simulink model "GalacticSoupFunctional"  (R2025b)
settings: Solver=VariableStepAuto  StartTime=0.0  StopTime=10.0  RelTol=1e-3
settings Model: DataDictionary=GalacticSoupFunctionalInterfaces.sldd  Creator=sarah  LastModifiedBy=sarah

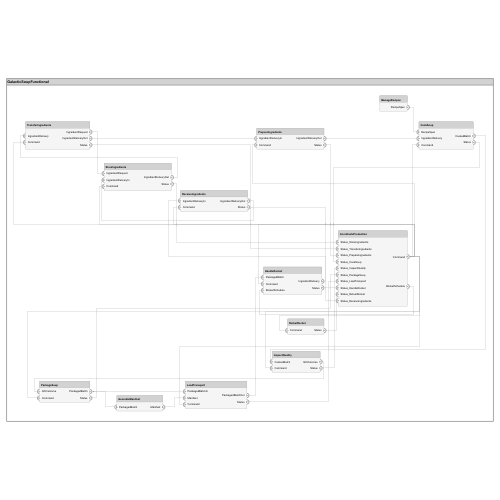
[thumbnail: Simulink's stored preview of the top-level diagram]
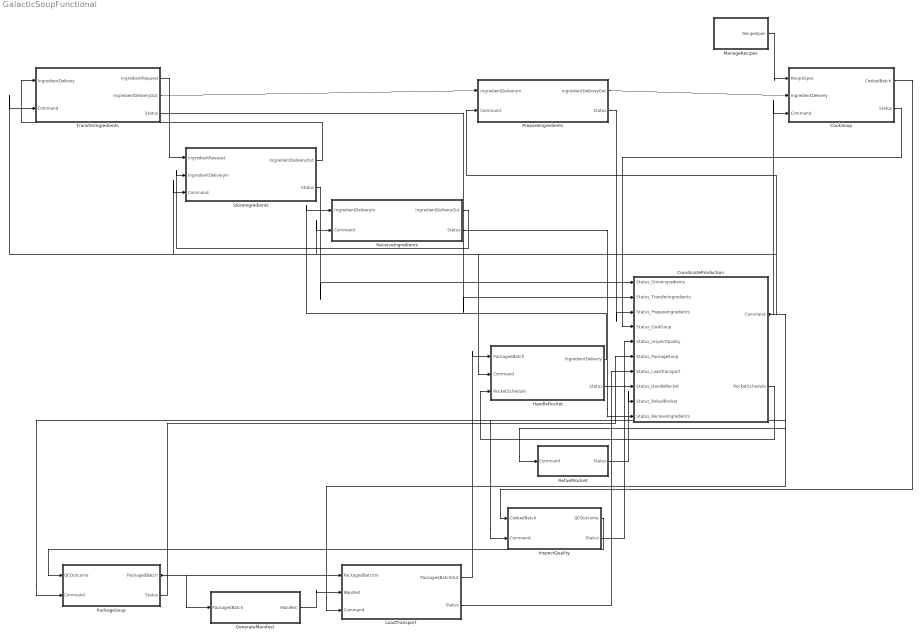
== system GalacticSoupFunctional ==
  CookSoup : Subsystem
      settings: PortSchema="{\"entries\":[{\"content\":{\"headerSize\":26,\"margin\":15,\"minimumSpacing\":25,\"sides\":[{\"content\":{\"connectorIds\":[\"In1\",\"In2\",\"In3\"]},\"type\":\"ConnectorPlacement.EquallySpacedRectSide\",\"uuid\":\"47548036-a6c3-440f-b573-2a4e753e82ae\"},{\"content\":{\"connectorIds\":[\"Out1\",\"Out2\"],\"side\":\"RIGHT\"},\"type\":\"ConnectorPlacement.EquallySpacedRectSide\",\"uuid\":\"ab096620-2054-4429-8520-52cfe6541bb8\"},{\"content\":{\"side\":\"TOP\"},\"type\":\"ConnectorPlacement.EquallySpacedRectSide\",\"uuid\":\"6e18e29c-ba68-48ca-8847-f496b38e15b5\"}]},\"type\":\"ConnectorPlacement.EquallySpacedConnector\",\"uuid\":\"7233fc04-a641-40d9-8870-909b934a9733\"}],\"packageUris\":[\"http://schema.mathworks.com/mf0/Connector/R2020b\"],\"version\":\"1.0\"}"
  CoordinateProduction : Subsystem
      settings: PortSchema="{\"entries\":[{\"content\":{\"headerSize\":26,\"margin\":15,\"minimumSpacing\":25,\"sides\":[{\"content\":{\"connectorIds\":[\"In1\",\"In2\",\"In3\",\"In4\",\"In5\",\"In6\",\"In7\",\"In8\",\"In9\",\"In10\"]},\"type\":\"ConnectorPlacement.EquallySpacedRectSide\",\"uuid\":\"47548036-a6c3-440f-b573-2a4e753e82ae\"},{\"content\":{\"connectorIds\":[\"Out1\",\"Out2\"],\"side\":\"RIGHT\"},\"type\":\"ConnectorPlacement.EquallySpacedRectSide\",\"uuid\":\"ab096620-2054-4429-8520-52cfe6541bb8\"},{\"content\":{\"side\":\"TOP\"},\"type\":\"ConnectorPlacement.EquallySpacedRectSide\",\"uuid\":\"6e18e29c-ba68-48ca-8847-f496b38e15b5\"}]},\"type\":\"ConnectorPlacement.EquallySpacedConnector\",\"uuid\":\"7233fc04-a641-40d9-8870-909b934a9733\"}],\"packageUris\":[\"http://schema.mathworks.com/mf0/Connector/R2020b\"],\"version\":\"1.0\"}"
  GenerateManifest : Subsystem
      settings: PortSchema="{\"entries\":[{\"content\":{\"headerSize\":26,\"margin\":15,\"minimumSpacing\":25,\"sides\":[{\"content\":{\"connectorIds\":[\"In1\"]},\"type\":\"ConnectorPlacement.EquallySpacedRectSide\",\"uuid\":\"47548036-a6c3-440f-b573-2a4e753e82ae\"},{\"content\":{\"connectorIds\":[\"Out1\"],\"side\":\"RIGHT\"},\"type\":\"ConnectorPlacement.EquallySpacedRectSide\",\"uuid\":\"ab096620-2054-4429-8520-52cfe6541bb8\"},{\"content\":{\"side\":\"TOP\"},\"type\":\"ConnectorPlacement.EquallySpacedRectSide\",\"uuid\":\"6e18e29c-ba68-48ca-8847-f496b38e15b5\"}]},\"type\":\"ConnectorPlacement.EquallySpacedConnector\",\"uuid\":\"7233fc04-a641-40d9-8870-909b934a9733\"}],\"packageUris\":[\"http://schema.mathworks.com/mf0/Connector/R2020b\"],\"version\":\"1.0\"}"
  HandleRocket : Subsystem
      settings: PortSchema="{\"entries\":[{\"content\":{\"headerSize\":26,\"margin\":15,\"minimumSpacing\":25,\"sides\":[{\"content\":{\"connectorIds\":[\"In1\",\"In2\",\"In3\"]},\"type\":\"ConnectorPlacement.EquallySpacedRectSide\",\"uuid\":\"47548036-a6c3-440f-b573-2a4e753e82ae\"},{\"content\":{\"connectorIds\":[\"Out1\",\"Out2\"],\"side\":\"RIGHT\"},\"type\":\"ConnectorPlacement.EquallySpacedRectSide\",\"uuid\":\"ab096620-2054-4429-8520-52cfe6541bb8\"},{\"content\":{\"side\":\"TOP\"},\"type\":\"ConnectorPlacement.EquallySpacedRectSide\",\"uuid\":\"6e18e29c-ba68-48ca-8847-f496b38e15b5\"}]},\"type\":\"ConnectorPlacement.EquallySpacedConnector\",\"uuid\":\"7233fc04-a641-40d9-8870-909b934a9733\"}],\"packageUris\":[\"http://schema.mathworks.com/mf0/Connector/R2020b\"],\"version\":\"1.0\"}"
  InspectQuality : Subsystem
      settings: PortSchema="{\"entries\":[{\"content\":{\"headerSize\":26,\"margin\":15,\"minimumSpacing\":25,\"sides\":[{\"content\":{\"connectorIds\":[\"In1\",\"In2\"]},\"type\":\"ConnectorPlacement.EquallySpacedRectSide\",\"uuid\":\"47548036-a6c3-440f-b573-2a4e753e82ae\"},{\"content\":{\"connectorIds\":[\"Out1\",\"Out2\"],\"side\":\"RIGHT\"},\"type\":\"ConnectorPlacement.EquallySpacedRectSide\",\"uuid\":\"ab096620-2054-4429-8520-52cfe6541bb8\"},{\"content\":{\"side\":\"TOP\"},\"type\":\"ConnectorPlacement.EquallySpacedRectSide\",\"uuid\":\"6e18e29c-ba68-48ca-8847-f496b38e15b5\"}]},\"type\":\"ConnectorPlacement.EquallySpacedConnector\",\"uuid\":\"7233fc04-a641-40d9-8870-909b934a9733\"}],\"packageUris\":[\"http://schema.mathworks.com/mf0/Connector/R2020b\"],\"version\":\"1.0\"}"
  LoadTransport : Subsystem
      settings: PortSchema="{\"entries\":[{\"content\":{\"headerSize\":26,\"margin\":15,\"minimumSpacing\":25,\"sides\":[{\"content\":{\"connectorIds\":[\"In1\",\"In2\",\"In3\"]},\"type\":\"ConnectorPlacement.EquallySpacedRectSide\",\"uuid\":\"47548036-a6c3-440f-b573-2a4e753e82ae\"},{\"content\":{\"connectorIds\":[\"Out1\",\"Out2\"],\"side\":\"RIGHT\"},\"type\":\"ConnectorPlacement.EquallySpacedRectSide\",\"uuid\":\"ab096620-2054-4429-8520-52cfe6541bb8\"},{\"content\":{\"side\":\"TOP\"},\"type\":\"ConnectorPlacement.EquallySpacedRectSide\",\"uuid\":\"6e18e29c-ba68-48ca-8847-f496b38e15b5\"}]},\"type\":\"ConnectorPlacement.EquallySpacedConnector\",\"uuid\":\"7233fc04-a641-40d9-8870-909b934a9733\"}],\"packageUris\":[\"http://schema.mathworks.com/mf0/Connector/R2020b\"],\"version\":\"1.0\"}"
  ManageRecipes : Subsystem
      settings: PortSchema="{\"entries\":[{\"content\":{\"headerSize\":26,\"margin\":15,\"minimumSpacing\":25,\"sides\":[{\"content\":{},\"type\":\"ConnectorPlacement.EquallySpacedRectSide\",\"uuid\":\"47548036-a6c3-440f-b573-2a4e753e82ae\"},{\"content\":{\"connectorIds\":[\"Out1\"],\"side\":\"RIGHT\"},\"type\":\"ConnectorPlacement.EquallySpacedRectSide\",\"uuid\":\"ab096620-2054-4429-8520-52cfe6541bb8\"},{\"content\":{\"side\":\"TOP\"},\"type\":\"ConnectorPlacement.EquallySpacedRectSide\",\"uuid\":\"6e18e29c-ba68-48ca-8847-f496b38e15b5\"}]},\"type\":\"ConnectorPlacement.EquallySpacedConnector\",\"uuid\":\"7233fc04-a641-40d9-8870-909b934a9733\"}],\"packageUris\":[\"http://schema.mathworks.com/mf0/Connector/R2020b\"],\"version\":\"1.0\"}"
  PackageSoup : Subsystem
      settings: PortSchema="{\"entries\":[{\"content\":{\"headerSize\":26,\"margin\":15,\"minimumSpacing\":25,\"sides\":[{\"content\":{\"connectorIds\":[\"In1\",\"In2\"]},\"type\":\"ConnectorPlacement.EquallySpacedRectSide\",\"uuid\":\"47548036-a6c3-440f-b573-2a4e753e82ae\"},{\"content\":{\"connectorIds\":[\"Out1\",\"Out2\"],\"side\":\"RIGHT\"},\"type\":\"ConnectorPlacement.EquallySpacedRectSide\",\"uuid\":\"ab096620-2054-4429-8520-52cfe6541bb8\"},{\"content\":{\"side\":\"TOP\"},\"type\":\"ConnectorPlacement.EquallySpacedRectSide\",\"uuid\":\"6e18e29c-ba68-48ca-8847-f496b38e15b5\"}]},\"type\":\"ConnectorPlacement.EquallySpacedConnector\",\"uuid\":\"7233fc04-a641-40d9-8870-909b934a9733\"}],\"packageUris\":[\"http://schema.mathworks.com/mf0/Connector/R2020b\"],\"version\":\"1.0\"}"
  PrepareIngredients : Subsystem
      settings: PortSchema="{\"entries\":[{\"content\":{\"headerSize\":26,\"margin\":15,\"minimumSpacing\":25,\"sides\":[{\"content\":{\"connectorIds\":[\"In1\",\"In2\"]},\"type\":\"ConnectorPlacement.EquallySpacedRectSide\",\"uuid\":\"47548036-a6c3-440f-b573-2a4e753e82ae\"},{\"content\":{\"connectorIds\":[\"Out1\",\"Out2\"],\"side\":\"RIGHT\"},\"type\":\"ConnectorPlacement.EquallySpacedRectSide\",\"uuid\":\"ab096620-2054-4429-8520-52cfe6541bb8\"},{\"content\":{\"side\":\"TOP\"},\"type\":\"ConnectorPlacement.EquallySpacedRectSide\",\"uuid\":\"6e18e29c-ba68-48ca-8847-f496b38e15b5\"}]},\"type\":\"ConnectorPlacement.EquallySpacedConnector\",\"uuid\":\"7233fc04-a641-40d9-8870-909b934a9733\"}],\"packageUris\":[\"http://schema.mathworks.com/mf0/Connector/R2020b\"],\"version\":\"1.0\"}"
  ReceiveIngredients : Subsystem
      settings: PortSchema="{\"entries\":[{\"content\":{\"headerSize\":26,\"margin\":15,\"minimumSpacing\":25,\"sides\":[{\"content\":{\"connectorIds\":[\"In1\",\"In2\"]},\"type\":\"ConnectorPlacement.EquallySpacedRectSide\",\"uuid\":\"47548036-a6c3-440f-b573-2a4e753e82ae\"},{\"content\":{\"connectorIds\":[\"Out1\",\"Out2\"],\"side\":\"RIGHT\"},\"type\":\"ConnectorPlacement.EquallySpacedRectSide\",\"uuid\":\"ab096620-2054-4429-8520-52cfe6541bb8\"},{\"content\":{\"side\":\"TOP\"},\"type\":\"ConnectorPlacement.EquallySpacedRectSide\",\"uuid\":\"6e18e29c-ba68-48ca-8847-f496b38e15b5\"}]},\"type\":\"ConnectorPlacement.EquallySpacedConnector\",\"uuid\":\"7233fc04-a641-40d9-8870-909b934a9733\"}],\"packageUris\":[\"http://schema.mathworks.com/mf0/Connector/R2020b\"],\"version\":\"1.0\"}"
  RefuelRocket : Subsystem
      settings: PortSchema="{\"entries\":[{\"content\":{\"headerSize\":26,\"margin\":15,\"minimumSpacing\":25,\"sides\":[{\"content\":{\"connectorIds\":[\"In1\"]},\"type\":\"ConnectorPlacement.EquallySpacedRectSide\",\"uuid\":\"47548036-a6c3-440f-b573-2a4e753e82ae\"},{\"content\":{\"connectorIds\":[\"Out1\"],\"side\":\"RIGHT\"},\"type\":\"ConnectorPlacement.EquallySpacedRectSide\",\"uuid\":\"ab096620-2054-4429-8520-52cfe6541bb8\"},{\"content\":{\"side\":\"TOP\"},\"type\":\"ConnectorPlacement.EquallySpacedRectSide\",\"uuid\":\"6e18e29c-ba68-48ca-8847-f496b38e15b5\"}]},\"type\":\"ConnectorPlacement.EquallySpacedConnector\",\"uuid\":\"7233fc04-a641-40d9-8870-909b934a9733\"}],\"packageUris\":[\"http://schema.mathworks.com/mf0/Connector/R2020b\"],\"version\":\"1.0\"}"
  StoreIngredients : Subsystem
      settings: PortSchema="{\"entries\":[{\"content\":{\"headerSize\":26,\"margin\":15,\"minimumSpacing\":25,\"sides\":[{\"content\":{\"connectorIds\":[\"In1\",\"In2\",\"In3\"]},\"type\":\"ConnectorPlacement.EquallySpacedRectSide\",\"uuid\":\"47548036-a6c3-440f-b573-2a4e753e82ae\"},{\"content\":{\"connectorIds\":[\"Out1\",\"Out2\"],\"side\":\"RIGHT\"},\"type\":\"ConnectorPlacement.EquallySpacedRectSide\",\"uuid\":\"ab096620-2054-4429-8520-52cfe6541bb8\"},{\"content\":{\"side\":\"TOP\"},\"type\":\"ConnectorPlacement.EquallySpacedRectSide\",\"uuid\":\"6e18e29c-ba68-48ca-8847-f496b38e15b5\"}]},\"type\":\"ConnectorPlacement.EquallySpacedConnector\",\"uuid\":\"7233fc04-a641-40d9-8870-909b934a9733\"}],\"packageUris\":[\"http://schema.mathworks.com/mf0/Connector/R2020b\"],\"version\":\"1.0\"}"
  TransferIngredients : Subsystem
      settings: PortSchema="{\"entries\":[{\"content\":{\"headerSize\":26,\"margin\":15,\"minimumSpacing\":25,\"sides\":[{\"content\":{\"connectorIds\":[\"In1\",\"In2\"]},\"type\":\"ConnectorPlacement.EquallySpacedRectSide\",\"uuid\":\"47548036-a6c3-440f-b573-2a4e753e82ae\"},{\"content\":{\"connectorIds\":[\"Out1\",\"Out2\",\"Out3\"],\"side\":\"RIGHT\"},\"type\":\"ConnectorPlacement.EquallySpacedRectSide\",\"uuid\":\"ab096620-2054-4429-8520-52cfe6541bb8\"},{\"content\":{\"side\":\"TOP\"},\"type\":\"ConnectorPlacement.EquallySpacedRectSide\",\"uuid\":\"6e18e29c-ba68-48ca-8847-f496b38e15b5\"}]},\"type\":\"ConnectorPlacement.EquallySpacedConnector\",\"uuid\":\"7233fc04-a641-40d9-8870-909b934a9733\"}],\"packageUris\":[\"http://schema.mathworks.com/mf0/Connector/R2020b\"],\"version\":\"1.0\"}"
  wires:
  GenerateManifest/1(Manifest) -> LoadTransport/2(Manifest)
  TransferIngredients/1(IngredientRequest) -> StoreIngredients/1(IngredientRequest)
  LoadTransport/1(PackagedBatchOut) -> HandleRocket/1(PackagedBatch)
  StoreIngredients/1(IngredientDeliveryOut) -> TransferIngredients/1(IngredientDelivery)
  TransferIngredients/2(IngredientDeliveryOut) -> PrepareIngredients/1(IngredientDeliveryIn)
  HandleRocket/2(Status) -> CoordinateProduction/8(Status_HandleRocket)
  TransferIngredients/3(Status) -> CoordinateProduction/2(Status_TransferIngredients)
  StoreIngredients/2(Status) -> CoordinateProduction/1(Status_StoreIngredients)
  PackageSoup/1(PackagedBatch) -> LoadTransport/1(PackagedBatchIn), GenerateManifest/1(PackagedBatch)
  PackageSoup/2(Status) -> CoordinateProduction/6(Status_PackageSoup)
  ReceiveIngredients/1(IngredientDeliveryOut) -> StoreIngredients/2(IngredientDeliveryIn)
  ReceiveIngredients/2(Status) -> CoordinateProduction/10(Status_ReceiveIngredients)
  InspectQuality/2(Status) -> CoordinateProduction/5(Status_InspectQuality)
  LoadTransport/2(Status) -> CoordinateProduction/7(Status_LoadTransport)
  PrepareIngredients/1(IngredientDeliveryOut) -> CookSoup/2(IngredientDelivery)
  PrepareIngredients/2(Status) -> CoordinateProduction/3(Status_PrepareIngredients)
  CookSoup/2(Status) -> CoordinateProduction/4(Status_CookSoup)
  ManageRecipes/1(RecipeSpec) -> CookSoup/1(RecipeSpec)
  HandleRocket/1(IngredientDelivery) -> ReceiveIngredients/1(IngredientDeliveryIn)
  RefuelRocket/1(Status) -> CoordinateProduction/9(Status_RefuelRocket)
  InspectQuality/1(QCOutcome) -> PackageSoup/1(QCOutcome)
  CoordinateProduction/1(Command) -> StoreIngredients/3(Command), TransferIngredients/2(Command), InspectQuality/2(Command), LoadTransport/3(Command), PackageSoup/2(Command), HandleRocket/2(Command), RefuelRocket/1(Command), ReceiveIngredients/2(Command), PrepareIngredients/2(Command), CookSoup/3(Command)
  CoordinateProduction/2(RocketSchedule) -> HandleRocket/3(RocketSchedule)
  CookSoup/1(CookedBatch) -> InspectQuality/1(CookedBatch)

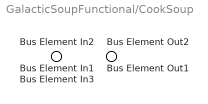
== system GalacticSoupFunctional/CookSoup ==
  Bus Element In1 : Inport  PortName=RecipeSpec
  Bus Element In2 : Inport  Port=2  PortName=IngredientDelivery
  Bus Element In3 : Inport  Port=3  PortName=Command
  Bus Element Out1 : Outport  PortName=CookedBatch
  Bus Element Out2 : Outport  Port=2  PortName=Status

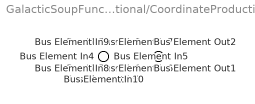
== system GalacticSoupFunctional/CoordinateProduction ==
  Bus Element In1 : Inport  PortName=Status_StoreIngredients
  Bus Element In2 : Inport  Port=2  PortName=Status_TransferIngredients
  Bus Element In3 : Inport  Port=3  PortName=Status_PrepareIngredients
  Bus Element In4 : Inport  Port=4  PortName=Status_CookSoup
  Bus Element In5 : Inport  Port=5  PortName=Status_InspectQuality
  Bus Element In6 : Inport  Port=6  PortName=Status_PackageSoup
  Bus Element In7 : Inport  Port=7  PortName=Status_LoadTransport
  Bus Element In8 : Inport  Port=8  PortName=Status_HandleRocket
  Bus Element In9 : Inport  Port=9  PortName=Status_RefuelRocket
  Bus Element In10 : Inport  Port=10  PortName=Status_ReceiveIngredients
  Bus Element Out1 : Outport  PortName=Command
  Bus Element Out2 : Outport  Port=2  PortName=RocketSchedule

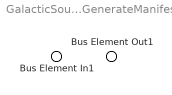
== system GalacticSoupFunctional/GenerateManifest ==
  Bus Element In1 : Inport  PortName=PackagedBatch
  Bus Element Out1 : Outport  PortName=Manifest

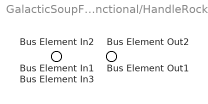
== system GalacticSoupFunctional/HandleRocket ==
  Bus Element In1 : Inport  PortName=PackagedBatch
  Bus Element In2 : Inport  Port=2  PortName=Command
  Bus Element In3 : Inport  Port=3  PortName=RocketSchedule
  Bus Element Out1 : Outport  PortName=IngredientDelivery
  Bus Element Out2 : Outport  Port=2  PortName=Status

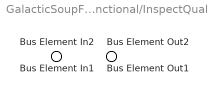
== system GalacticSoupFunctional/InspectQuality ==
  Bus Element In1 : Inport  PortName=CookedBatch
  Bus Element In2 : Inport  Port=2  PortName=Command
  Bus Element Out1 : Outport  PortName=QCOutcome
  Bus Element Out2 : Outport  Port=2  PortName=Status

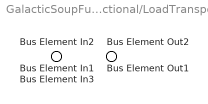
== system GalacticSoupFunctional/LoadTransport ==
  Bus Element In1 : Inport  PortName=PackagedBatchIn
  Bus Element In2 : Inport  Port=2  PortName=Manifest
  Bus Element In3 : Inport  Port=3  PortName=Command
  Bus Element Out1 : Outport  PortName=PackagedBatchOut
  Bus Element Out2 : Outport  Port=2  PortName=Status

== system GalacticSoupFunctional/ManageRecipes ==
  Bus Element Out1 : Outport  PortName=RecipeSpec

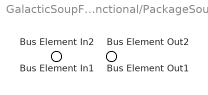
== system GalacticSoupFunctional/PackageSoup ==
  Bus Element In1 : Inport  PortName=QCOutcome
  Bus Element In2 : Inport  Port=2  PortName=Command
  Bus Element Out1 : Outport  PortName=PackagedBatch
  Bus Element Out2 : Outport  Port=2  PortName=Status

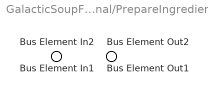
== system GalacticSoupFunctional/PrepareIngredients ==
  Bus Element In1 : Inport  PortName=IngredientDeliveryIn
  Bus Element In2 : Inport  Port=2  PortName=Command
  Bus Element Out1 : Outport  PortName=IngredientDeliveryOut
  Bus Element Out2 : Outport  Port=2  PortName=Status

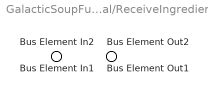
== system GalacticSoupFunctional/ReceiveIngredients ==
  Bus Element In1 : Inport  PortName=IngredientDeliveryIn
  Bus Element In2 : Inport  Port=2  PortName=Command
  Bus Element Out1 : Outport  PortName=IngredientDeliveryOut
  Bus Element Out2 : Outport  Port=2  PortName=Status

== system GalacticSoupFunctional/RefuelRocket ==
  Bus Element In1 : Inport  PortName=Command
  Bus Element Out1 : Outport  PortName=Status

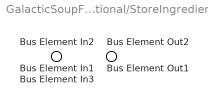
== system GalacticSoupFunctional/StoreIngredients ==
  Bus Element In1 : Inport  PortName=IngredientRequest
  Bus Element In2 : Inport  Port=2  PortName=IngredientDeliveryIn
  Bus Element In3 : Inport  Port=3  PortName=Command
  Bus Element Out1 : Outport  PortName=IngredientDeliveryOut
  Bus Element Out2 : Outport  Port=2  PortName=Status

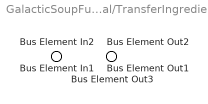
== system GalacticSoupFunctional/TransferIngredients ==
  Bus Element In1 : Inport  PortName=IngredientDelivery
  Bus Element In2 : Inport  Port=2  PortName=Command
  Bus Element Out1 : Outport  PortName=IngredientRequest
  Bus Element Out2 : Outport  Port=2  PortName=IngredientDeliveryOut
  Bus Element Out3 : Outport  Port=3  PortName=Status
